simulink subsystem "RobotPlant"  (R2022b)
settings: Solver=VariableStepAuto  StartTime=0.0  StopTime=10.0  RelTol=1e-3
settings Model: Creator=Sahil Gaurkar  LastModifiedBy=Sahil Gaurkar

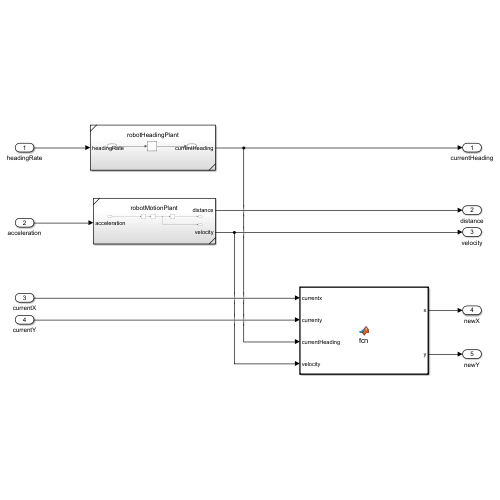
[thumbnail: Simulink's stored preview of the top-level diagram]
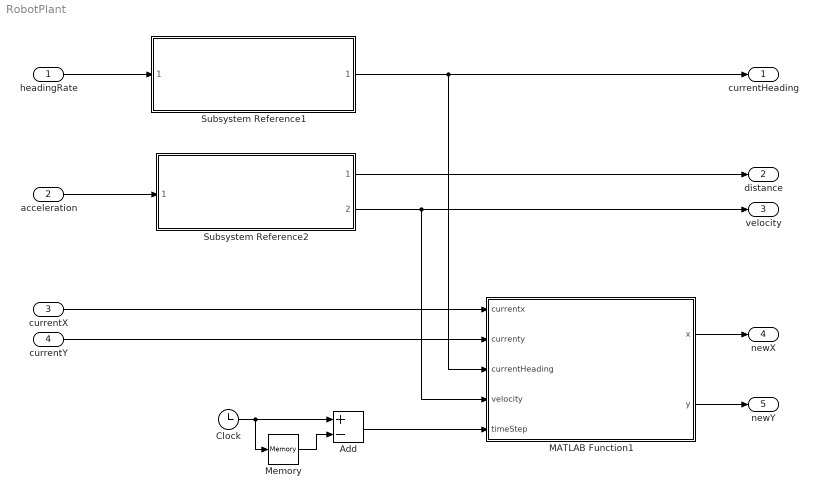
== system RobotPlant ==
  headingRate : Inport
  acceleration : Inport  Port=2
  currentX : Inport  Port=3
  currentY : Inport  Port=4
  Add : Sum  Inputs=+-
  Clock : Clock
  MATLAB Function1 : MATLAB Function  TreatAsAtomicUnit=on
  Memory : Memory
  Subsystem Reference1 : Subsystem  ReferencedSubsystem=robotHeadingPlant
  Subsystem Reference2 : Subsystem  ReferencedSubsystem=robotMotionPlant
  currentHeading : Outport
  distance : Outport  Port=2
  velocity : Outport  Port=3
  newX : Outport  Port=4
  newY : Outport  Port=5
  wires:
  headingRate/1 -> Subsystem Reference1/1
  acceleration/1 -> Subsystem Reference2/1
  Subsystem Reference2/2 -> MATLAB Function1/4(velocity), velocity/1
  Subsystem Reference2/1 -> distance/1
  Subsystem Reference1/1 -> MATLAB Function1/3(currentHeading), currentHeading/1
  currentY/1 -> MATLAB Function1/2(currenty)
  currentX/1 -> MATLAB Function1/1(currentx)
  MATLAB Function1/1(x) -> newX/1
  MATLAB Function1/2(y) -> newY/1
  Clock/1 -> Add/1, Memory/1
  Memory/1 -> Add/2
  Add/1 -> MATLAB Function1/5(timeStep)

== matlab function RobotPlant/MATLAB Function1 ==
  data: currentx input; currenty input; currentHeading input; x output; velocity input; y output; timeStep input
function [x,y]  = fcn(currentx, currenty, currentHeading, velocity, timeStep)


x = currentx + velocity * cosd(currentHeading) * timeStep;
y = currenty + velocity * sind(currentHeading)* timeStep;
